simulink library "LopesDevelopmentLibrary"  (R2015b)
settings: Solver=ode45  StartTime=0.0  StopTime=10.0  RelTol=1e-3
values from neighbouring files (symbols this model uses):
  d2r = @(d) d*(pi/180)    [LopesDevelopmentLibrary_LoadParameters.m]
  ts = LopesParams.ts    [LopesDevelopmentLibrary_LoadParameters.m]
undefined symbols (not defined in the file or in its folder): anyParameterChanged, DiscIntNeverNeededParam, gcbh, LAP, LHF, LKF, LopesParams, macaddr, mxpcnetworkconfig, mxpcrtudprx, mxpcrtudptx, patientParametersChanged, port, PX, PZ, RAP, RHF, RKF, SelectorLOPESInSize, StrideTime_s, Time
undefined symbols (not defined in the file): LopesParamsSendDataArrayLen
libraries: LopesDevelopmentLibrary x327, simulink x100, dspmtrx3 x49, xpciplib x6, xpcnetworkbufferlib x5, dspsigops x4, dspstat3 x3, xpcethernetlib x2, visionstatistics x2, xpcseriallib x2, LopesDevelopmentLibraryTest x1, nmc x1
(part 5 of 12)

== system LopesDevelopmentLibrary/GaitGeneration/CalculateReferenceStiffnesses/RHA1 ==
  General_GuidanceForce : Inport
  breaks : Inport  Port=2
  phase : Inport  Port=3
  WeightShift_GuidanceForce : Inport  Port=4
  Circumduction_GuidanceForce : Inport  Port=5
  CalculateStiffnessForOneJoint : LopesDevelopmentLibrary/BlocksForInternalUse/GaitGeneration/CalculateStiffnessForOneJoint
  Constant : Constant  Value=LopesParams.GaitData.StiffnessParameters.HA_WeightShift
  Constant1 : Constant  Value=LopesParams.GaitData.StiffnessParameters.HA_Circumduction
  Mux : Mux  Inputs=2
  Mux1 : Mux  Inputs=2
  TrajectoryOfInfluence : LopesDevelopmentLibrary/BlocksForInternalUse/GaitGeneration/TrajectoryOfInfluence
  TrajectoryOfInfluence1 : LopesDevelopmentLibrary/BlocksForInternalUse/GaitGeneration/TrajectoryOfInfluence
  Stiffness_pct : Outport
  wires:
  Mux1/1 -> CalculateStiffnessForOneJoint/3
  Mux/1 -> CalculateStiffnessForOneJoint/2
  Circumduction_GuidanceForce/1 -> Mux1/2
  TrajectoryOfInfluence1/1 -> Mux/2
  TrajectoryOfInfluence/1 -> Mux/1
  phase/1 -> TrajectoryOfInfluence1/3, TrajectoryOfInfluence/3
  breaks/1 -> TrajectoryOfInfluence1/2, TrajectoryOfInfluence/2
  Constant/1 -> TrajectoryOfInfluence/1
  WeightShift_GuidanceForce/1 -> Mux1/1
  Constant1/1 -> TrajectoryOfInfluence1/1
  General_GuidanceForce/1 -> CalculateStiffnessForOneJoint/1
  CalculateStiffnessForOneJoint/1 -> Stiffness_pct/1

== system LopesDevelopmentLibrary/GaitGeneration/CalculateReferenceStiffnesses/RHF ==
  General_GuidanceForce : Inport
  breaks : Inport  Port=2
  phase : Inport  Port=3
  FootPlacement_GuidanceForce : Inport  Port=4
  StepLength_GuidanceForce : Inport  Port=5
  CalculateStiffnessForOneJoint : LopesDevelopmentLibrary/BlocksForInternalUse/GaitGeneration/CalculateStiffnessForOneJoint
  Constant : Constant  Value=LopesParams.GaitData.StiffnessParameters.HF_FootPlacement
  Constant1 : Constant  Value=LopesParams.GaitData.StiffnessParameters.HF_StepLength
  Mux : Mux  Inputs=2
  Mux1 : Mux  Inputs=2
  TrajectoryOfInfluence : LopesDevelopmentLibrary/BlocksForInternalUse/GaitGeneration/TrajectoryOfInfluence
  TrajectoryOfInfluence1 : LopesDevelopmentLibrary/BlocksForInternalUse/GaitGeneration/TrajectoryOfInfluence
  Stiffness_pct : Outport
  wires:
  phase/1 -> TrajectoryOfInfluence1/3, TrajectoryOfInfluence/3
  breaks/1 -> TrajectoryOfInfluence1/2, TrajectoryOfInfluence/2
  Constant/1 -> TrajectoryOfInfluence/1
  FootPlacement_GuidanceForce/1 -> Mux1/1
  CalculateStiffnessForOneJoint/1 -> Stiffness_pct/1
  Constant1/1 -> TrajectoryOfInfluence1/1
  StepLength_GuidanceForce/1 -> Mux1/2
  TrajectoryOfInfluence/1 -> Mux/1
  TrajectoryOfInfluence1/1 -> Mux/2
  Mux/1 -> CalculateStiffnessForOneJoint/2
  Mux1/1 -> CalculateStiffnessForOneJoint/3
  General_GuidanceForce/1 -> CalculateStiffnessForOneJoint/1

== system LopesDevelopmentLibrary/GaitGeneration/CalculateReferenceStiffnesses/RKF ==
  General_GuidanceForce : Inport
  breaks : Inport  Port=2
  phase : Inport  Port=3
  StepHeight_GuidanceForce : Inport  Port=4
  StabilityInStance_GuidanceForce : Inport  Port=5
  FootPlacement_GuidanceForce : Inport  Port=6
  CalculateStiffnessForOneJoint : LopesDevelopmentLibrary/BlocksForInternalUse/GaitGeneration/CalculateStiffnessForOneJoint
  Constant : Constant  Value=LopesParams.GaitData.StiffnessParameters.KF_StepHeight
  Constant1 : Constant  Value=LopesParams.GaitData.StiffnessParameters.KF_StabilityStance
  Constant2 : Constant  Value=LopesParams.GaitData.StiffnessParameters.KF_FootPlacement
  Mux : Mux  Inputs=3
  Mux1 : Mux  Inputs=3
  TrajectoryOfInfluence : LopesDevelopmentLibrary/BlocksForInternalUse/GaitGeneration/TrajectoryOfInfluence
  TrajectoryOfInfluence1 : LopesDevelopmentLibrary/BlocksForInternalUse/GaitGeneration/TrajectoryOfInfluence
  TrajectoryOfInfluence2 : LopesDevelopmentLibrary/BlocksForInternalUse/GaitGeneration/TrajectoryOfInfluence
  Stiffness_pct : Outport
  wires:
  StabilityInStance_GuidanceForce/1 -> Mux1/2
  Constant1/1 -> TrajectoryOfInfluence1/1
  TrajectoryOfInfluence1/1 -> Mux/2
  TrajectoryOfInfluence/1 -> Mux/1
  StepHeight_GuidanceForce/1 -> Mux1/1
  Constant/1 -> TrajectoryOfInfluence/1
  breaks/1 -> TrajectoryOfInfluence/2, TrajectoryOfInfluence2/2, TrajectoryOfInfluence1/2
  phase/1 -> TrajectoryOfInfluence/3, TrajectoryOfInfluence2/3, TrajectoryOfInfluence1/3
  FootPlacement_GuidanceForce/1 -> Mux1/3
  Constant2/1 -> TrajectoryOfInfluence2/1
  TrajectoryOfInfluence2/1 -> Mux/3
  CalculateStiffnessForOneJoint/1 -> Stiffness_pct/1
  Mux/1 -> CalculateStiffnessForOneJoint/2
  Mux1/1 -> CalculateStiffnessForOneJoint/3
  General_GuidanceForce/1 -> CalculateStiffnessForOneJoint/1

== system LopesDevelopmentLibrary/GaitGeneration/GaitParameters/AssignChangedElements ==
  note: This block checks whether any of the parameters changed during
      | this sampletime, and assigns the correct values to the anyParameterChanged
      | and patientParametersChanged bus elements.
  BusIn : Inport
  PatientParametersChanged : Inport  Port=2
  AnyChanged : LopesDevelopmentLibrary/Various/AnyChanged
  Bus Assignment : BusAssignment  AssignedSignals=patientParametersChanged,anyParameterChanged
  Bus Selector : BusSelector  OutputSignals=Patient,General,WeightShift,LeftStepHeight,RightStepHeight,LeftCircumduction,RightCircumduction,LeftStabilityStance,RightStabilityStance,LeftPrepositioning,RightPrepositioning,LeftSteplength,RightSteplength  OutputAsBus=on
  Data Type Conversion2 : DataTypeConversion
  Logical Operator : Logic  Operator=OR  AllPortsSameDT=off  OutDataTypeStr=boolean
  BusOut : Outport
  Changed : Outport  Port=2
  wires:
  Data Type Conversion2/1 -> Changed/1
  Bus Assignment/1 -> BusOut/1
  Bus Selector/1 -> AnyChanged/1
  PatientParametersChanged/1 -> Logical Operator/1, Bus Assignment/2
  BusIn/1 -> Bus Selector/1, Bus Assignment/1
  Logical Operator/1 -> Bus Assignment/3, Data Type Conversion2/1
  AnyChanged/1 -> Logical Operator/2

== system LopesDevelopmentLibrary/GaitGeneration/GaitParameters/Circumduction ==

== system LopesDevelopmentLibrary/GaitGeneration/GaitParameters/General ==

== system LopesDevelopmentLibrary/GaitGeneration/GaitParameters/Prepositioning ==

== system LopesDevelopmentLibrary/GaitGeneration/GaitParameters/Pushoff ==

== system LopesDevelopmentLibrary/GaitGeneration/GaitParameters/RateLimitCircumduction ==
  GeneralGF : Inport
  In2 : Inport  Port=2
  In3 : Inport  Port=3
  In4 : Inport  Port=4
  In5 : Inport  Port=5
  In6 : Inport  Port=6
  In7 : Inport  Port=7
  Bus Creator1 : BusCreator  Inputs=2
  Bus Creator2 : BusCreator  Inputs=2
  Rate Limiter : RateLimiter  RisingSlewLimit=100  FallingSlewLimit=-100  SampleTimeMode=inherited
  Rate Limiter1 : RateLimiter  RisingSlewLimit=50  FallingSlewLimit=-50  SampleTimeMode=inherited
  Rate Limiter2 : RateLimiter  RisingSlewLimit=50  FallingSlewLimit=-50  SampleTimeMode=inherited
  Rate Limiter7 : RateLimiter  RisingSlewLimit=100  FallingSlewLimit=-100  SampleTimeMode=inherited
  Switch : Switch  Criteria=u2 ~= 0
  Switch1 : Switch  Criteria=u2 ~= 0
  Left : Outport
  Right : Outport  Port=2
  wires:
  Bus Creator1/1 -> Left/1
  Rate Limiter1/1 -> Bus Creator1/2  "Circumduction_pct"
  Rate Limiter/1 -> Bus Creator1/1  "GuidanceForce_pct"
  Switch1/1 -> Rate Limiter7/1
  In2/1 -> Switch/2
  In6/1 -> Switch1/1
  In3/1 -> Switch/1
  In5/1 -> Switch1/2
  In7/1 -> Rate Limiter2/1
  Switch/1 -> Rate Limiter/1  "GuidanceForce_pct"
  In4/1 -> Rate Limiter1/1
  GeneralGF/1 -> Switch/3, Switch1/3
  Rate Limiter2/1 -> Bus Creator2/2  "Circumduction_pct"
  Rate Limiter7/1 -> Bus Creator2/1  "GuidanceForce_pct"
  Bus Creator2/1 -> Right/1

== system LopesDevelopmentLibrary/GaitGeneration/GaitParameters/RateLimitGeneral ==
  In1 : Inport
  In2 : Inport  Port=2
  In3 : Inport  Port=3
  Bus Creator1 : BusCreator  Inputs=3
  ConvertToKm_h : Gain  Gain=3.6
  Rate Limiter1 : RateLimiter  RisingSlewLimit=50  FallingSlewLimit=-50  SampleTimeMode=inherited
  Rate Limiter2 : RateLimiter  RisingSlewLimit=0.1  FallingSlewLimit=-0.1  SampleTimeMode=inherited
  Rate Limiter3 : RateLimiter  RisingSlewLimit=20  FallingSlewLimit=-20  SampleTimeMode=inherited
  km_h : Outport
  General : Outport  Port=2
  wires:
  Bus Creator1/1 -> General/1  "General"
  In3/1 -> Rate Limiter1/1
  In2/1 -> Rate Limiter3/1
  In1/1 -> ConvertToKm_h/1, Rate Limiter2/1
  ConvertToKm_h/1 -> km_h/1
  Rate Limiter2/1 -> Bus Creator1/1  "WalkingVelocity_m_s"
  Rate Limiter3/1 -> Bus Creator1/2  "GuidanceForce_pct"
  Rate Limiter1/1 -> Bus Creator1/3  "HipExtensionOffset"

== system LopesDevelopmentLibrary/GaitGeneration/GaitParameters/RateLimitPrepositioning ==
  GeneralGF : Inport
  In2 : Inport  Port=2
  In3 : Inport  Port=3
  In4 : Inport  Port=4
  In1 : Inport  Port=5
  In5 : Inport  Port=6
  In6 : Inport  Port=7
  In7 : Inport  Port=8
  In8 : Inport  Port=9
  Bus Creator1 : BusCreator  Inputs=3
  Bus Creator2 : BusCreator  Inputs=3
  Rate Limiter : RateLimiter  RisingSlewLimit=100  FallingSlewLimit=-100  SampleTimeMode=inherited
  Rate Limiter{1..4} (4 alike) : RateLimiter  RisingSlewLimit=50  FallingSlewLimit=-50  SampleTimeMode=inherited
  Rate Limiter7 : RateLimiter  RisingSlewLimit=100  FallingSlewLimit=-100  SampleTimeMode=inherited
  Switch : Switch  Criteria=u2 ~= 0
  Switch1 : Switch  Criteria=u2 ~= 0
  Left : Outport
  Right : Outport  Port=2
  wires:
  Bus Creator1/1 -> Left/1
  Rate Limiter1/1 -> Bus Creator1/2  "KneeFlexion_pct"
  Rate Limiter/1 -> Bus Creator1/1  "GuidanceForce_pct"
  Switch1/1 -> Rate Limiter7/1
  In2/1 -> Switch/2
  In6/1 -> Switch1/1
  In3/1 -> Switch/1
  In5/1 -> Switch1/2
  In7/1 -> Rate Limiter2/1
  Switch/1 -> Rate Limiter/1  "GuidanceForce_pct"
  In4/1 -> Rate Limiter1/1
  GeneralGF/1 -> Switch/3, Switch1/3
  Rate Limiter2/1 -> Bus Creator2/2  "KneeFlexion_pct"
  Rate Limiter7/1 -> Bus Creator2/1  "GuidanceForce_pct"
  Bus Creator2/1 -> Right/1
  Rate Limiter3/1 -> Bus Creator1/3  "AnkleDorsiflexion_pct"
  In1/1 -> Rate Limiter3/1
  Rate Limiter4/1 -> Bus Creator2/3  "AnkleDorsiflexion_pct"
  In8/1 -> Rate Limiter4/1

== system LopesDevelopmentLibrary/GaitGeneration/GaitParameters/RateLimitPushoff ==
  GeneralGF : Inport
  In2 : Inport  Port=2
  In3 : Inport  Port=3
  In4 : Inport  Port=4
  In1 : Inport  Port=5
  In5 : Inport  Port=6
  In6 : Inport  Port=7
  In7 : Inport  Port=8
  In8 : Inport  Port=9
  Bus Creator1 : BusCreator  Inputs=3
  Bus Creator2 : BusCreator  Inputs=3
  Rate Limiter : RateLimiter  RisingSlewLimit=100  FallingSlewLimit=-100  SampleTimeMode=inherited
  Rate Limiter1 : RateLimiter  RisingSlewLimit=50  FallingSlewLimit=-50  SampleTimeMode=inherited
  Rate Limiter2 : RateLimiter  RisingSlewLimit=50  FallingSlewLimit=-50  SampleTimeMode=inherited
  Rate Limiter3 : RateLimiter  RisingSlewLimit=10  FallingSlewLimit=-10  SampleTimeMode=inherited
  Rate Limiter4 : RateLimiter  RisingSlewLimit=10  FallingSlewLimit=-10  SampleTimeMode=inherited
  Rate Limiter7 : RateLimiter  RisingSlewLimit=100  FallingSlewLimit=-100  SampleTimeMode=inherited
  Switch : Switch  Criteria=u2 ~= 0
  Switch1 : Switch  Criteria=u2 ~= 0
  Left : Outport
  Right : Outport  Port=2
  wires:
  In8/1 -> Rate Limiter4/1
  Rate Limiter4/1 -> Bus Creator2/3  "Timing_pct"
  In1/1 -> Rate Limiter3/1
  Rate Limiter3/1 -> Bus Creator1/3  "Timing_pct"
  Bus Creator2/1 -> Right/1
  Rate Limiter7/1 -> Bus Creator2/1  "GuidanceForce_pct"
  Rate Limiter2/1 -> Bus Creator2/2  "HipExtension_pct"
  GeneralGF/1 -> Switch1/3, Switch/3
  In4/1 -> Rate Limiter1/1
  Switch/1 -> Rate Limiter/1  "GuidanceForce_pct"
  In7/1 -> Rate Limiter2/1
  In5/1 -> Switch1/2
  In3/1 -> Switch/1
  In6/1 -> Switch1/1
  In2/1 -> Switch/2
  Switch1/1 -> Rate Limiter7/1
  Rate Limiter/1 -> Bus Creator1/1  "GuidanceForce_pct"
  Rate Limiter1/1 -> Bus Creator1/2  "HipExtension_pct"
  Bus Creator1/1 -> Left/1

== system LopesDevelopmentLibrary/GaitGeneration/GaitParameters/RateLimitStabilityStance ==
  GeneralGF : Inport
  In2 : Inport  Port=2
  In3 : Inport  Port=3
  In4 : Inport  Port=4
  In5 : Inport  Port=5
  In6 : Inport  Port=6
  In7 : Inport  Port=7
  Bus Creator1 : BusCreator  Inputs=2
  Bus Creator2 : BusCreator  Inputs=2
  Rate Limiter : RateLimiter  RisingSlewLimit=100  FallingSlewLimit=-100  SampleTimeMode=inherited
  Rate Limiter1 : RateLimiter  RisingSlewLimit=50  FallingSlewLimit=-50  SampleTimeMode=inherited
  Rate Limiter2 : RateLimiter  RisingSlewLimit=50  FallingSlewLimit=-50  SampleTimeMode=inherited
  Rate Limiter7 : RateLimiter  RisingSlewLimit=100  FallingSlewLimit=-100  SampleTimeMode=inherited
  Switch : Switch  Criteria=u2 ~= 0
  Switch1 : Switch  Criteria=u2 ~= 0
  Left : Outport
  Right : Outport  Port=2
  wires:
  Bus Creator2/1 -> Right/1
  Rate Limiter7/1 -> Bus Creator2/1  "GuidanceForce_pct"
  Rate Limiter2/1 -> Bus Creator2/2  "KneeFlexion_pct"
  GeneralGF/1 -> Switch1/3, Switch/3
  In4/1 -> Rate Limiter1/1
  Switch/1 -> Rate Limiter/1  "GuidanceForce_pct"
  In7/1 -> Rate Limiter2/1
  In5/1 -> Switch1/2
  In3/1 -> Switch/1
  In6/1 -> Switch1/1
  In2/1 -> Switch/2
  Switch1/1 -> Rate Limiter7/1
  Rate Limiter/1 -> Bus Creator1/1  "GuidanceForce_pct"
  Rate Limiter1/1 -> Bus Creator1/2  "KneeFlexion_pct"
  Bus Creator1/1 -> Left/1

== system LopesDevelopmentLibrary/GaitGeneration/GaitParameters/RateLimitStepHeight ==
  GeneralGF : Inport
  In2 : Inport  Port=2
  In3 : Inport  Port=3
  In1 : Inport  Port=4
  In4 : Inport  Port=5
  In5 : Inport  Port=6
  In6 : Inport  Port=7
  In8 : Inport  Port=8
  In7 : Inport  Port=9
  Bus Creator1 : BusCreator  Inputs=3
  Bus Creator2 : BusCreator  Inputs=3
  Rate Limiter : RateLimiter  RisingSlewLimit=100  FallingSlewLimit=-100  SampleTimeMode=inherited
  Rate Limiter1 : RateLimiter  RisingSlewLimit=50  FallingSlewLimit=-50  SampleTimeMode=inherited
  Rate Limiter2 : RateLimiter  RisingSlewLimit=50  FallingSlewLimit=-50  SampleTimeMode=inherited
  Rate Limiter3 : RateLimiter  RisingSlewLimit=100  FallingSlewLimit=-100  SampleTimeMode=inherited
  Rate Limiter4 : RateLimiter  RisingSlewLimit=50  FallingSlewLimit=-50  SampleTimeMode=inherited
  Rate Limiter7 : RateLimiter  RisingSlewLimit=100  FallingSlewLimit=-100  SampleTimeMode=inherited
  Switch : Switch  Criteria=u2 ~= 0
  Switch1 : Switch  Criteria=u2 ~= 0
  Left : Outport
  Right : Outport  Port=2
  wires:
  Bus Creator2/1 -> Right/1
  Rate Limiter7/1 -> Bus Creator2/1  "GuidanceForce_pct"
  Rate Limiter2/1 -> Bus Creator2/3  "KneeFlexion_pct"
  GeneralGF/1 -> Switch/3, Switch1/3
  In4/1 -> Rate Limiter1/1
  Switch/1 -> Rate Limiter/1  "GuidanceForce_pct"
  In7/1 -> Rate Limiter2/1
  In5/1 -> Switch1/2
  In3/1 -> Switch/1
  In6/1 -> Switch1/1
  In2/1 -> Switch/2
  Switch1/1 -> Rate Limiter7/1
  Rate Limiter/1 -> Bus Creator1/1  "GuidanceForce_pct"
  Rate Limiter1/1 -> Bus Creator1/3  "KneeFlexion_pct"
  Bus Creator1/1 -> Left/1
  Rate Limiter3/1 -> Bus Creator1/2  "AnkleDorsiflexion_pct"
  In1/1 -> Rate Limiter3/1
  Rate Limiter4/1 -> Bus Creator2/2  "AnkleDorsiflexion_pct"
  In8/1 -> Rate Limiter4/1

== system LopesDevelopmentLibrary/GaitGeneration/GaitParameters/RateLimitStepLength ==
  GeneralGF : Inport
  In2 : Inport  Port=2
  In3 : Inport  Port=3
  In4 : Inport  Port=4
  Bus Creator1 : BusCreator  Inputs=2
  Rate Limiter : RateLimiter  RisingSlewLimit=100  FallingSlewLimit=-100  SampleTimeMode=inherited
  Rate Limiter1 : RateLimiter  RisingSlewLimit=5  FallingSlewLimit=-5  SampleTimeMode=inherited
  Switch : Switch  Criteria=u2 ~= 0
  StepLength : Outport
  wires:
  GeneralGF/1 -> Switch/3
  In4/1 -> Rate Limiter1/1
  Switch/1 -> Rate Limiter/1  "GuidanceForce_pct"
  In3/1 -> Switch/1
  In2/1 -> Switch/2
  Rate Limiter/1 -> Bus Creator1/1  "GuidanceForce_pct"
  Rate Limiter1/1 -> Bus Creator1/2  "StepLength_pct"
  Bus Creator1/1 -> StepLength/1

== system LopesDevelopmentLibrary/GaitGeneration/GaitParameters/RateLimitWeightShift ==
  GeneralGF : Inport
  In2 : Inport  Port=2
  In3 : Inport  Port=3
  In4 : Inport  Port=4
  In5 : Inport  Port=5
  In6 : Inport  Port=6
  In7 : Inport  Port=7
  In8 : Inport  Port=8
  In9 : Inport  Port=9
  Bus Creator1 : BusCreator  Inputs=7
  Rate Limiter : RateLimiter  RisingSlewLimit=50  FallingSlewLimit=-50  SampleTimeMode=inherited
  Rate Limiter1 : RateLimiter  RisingSlewLimit=50  FallingSlewLimit=-50  SampleTimeMode=inherited
  Rate Limiter2 : RateLimiter  RisingSlewLimit=50  FallingSlewLimit=-50  SampleTimeMode=inherited
  Rate Limiter3 : RateLimiter  RisingSlewLimit=15  FallingSlewLimit=-15  SampleTimeMode=inherited
  Rate Limiter4 : RateLimiter  RisingSlewLimit=15  FallingSlewLimit=-15  SampleTimeMode=inherited
  Rate Limiter5 : RateLimiter  RisingSlewLimit=15  FallingSlewLimit=-15  SampleTimeMode=inherited
  Rate Limiter6 : RateLimiter  RisingSlewLimit=20  FallingSlewLimit=-20  SampleTimeMode=inherited
  Switch : Switch  Criteria=u2 ~= 0
  Out1 : Outport
  wires:
  In3/1 -> Switch/1
  Switch/1 -> Rate Limiter/1  "GuidanceForce_pct"
  In7/1 -> Rate Limiter4/1
  In8/1 -> Rate Limiter5/1
  In9/1 -> Rate Limiter6/1
  In4/1 -> Rate Limiter1/1
  In5/1 -> Rate Limiter2/1
  In6/1 -> Rate Limiter3/1
  GeneralGF/1 -> Switch/3
  Rate Limiter5/1 -> Bus Creator1/6  "DurationRight_pct"
  Rate Limiter/1 -> Bus Creator1/1  "GuidanceForce_pct"
  Rate Limiter4/1 -> Bus Creator1/5  "DurationLeft_pct"
  Rate Limiter3/1 -> Bus Creator1/4  "Timing_pct"
  Rate Limiter1/1 -> Bus Creator1/2  "AmplitudeLeft_pct"
  Rate Limiter6/1 -> Bus Creator1/7  "StepWidth_pct"
  Bus Creator1/1 -> Out1/1
  Rate Limiter2/1 -> Bus Creator1/3  "AmplitudeRight_pct"
  In2/1 -> Switch/2

== system LopesDevelopmentLibrary/GaitGeneration/GaitParameters/StabilityInStance ==

== system LopesDevelopmentLibrary/GaitGeneration/GaitParameters/StepHeight ==

== system LopesDevelopmentLibrary/GaitGeneration/GaitParameters/StepLength ==

== system LopesDevelopmentLibrary/GaitGeneration/GaitParameters/WeightShift ==

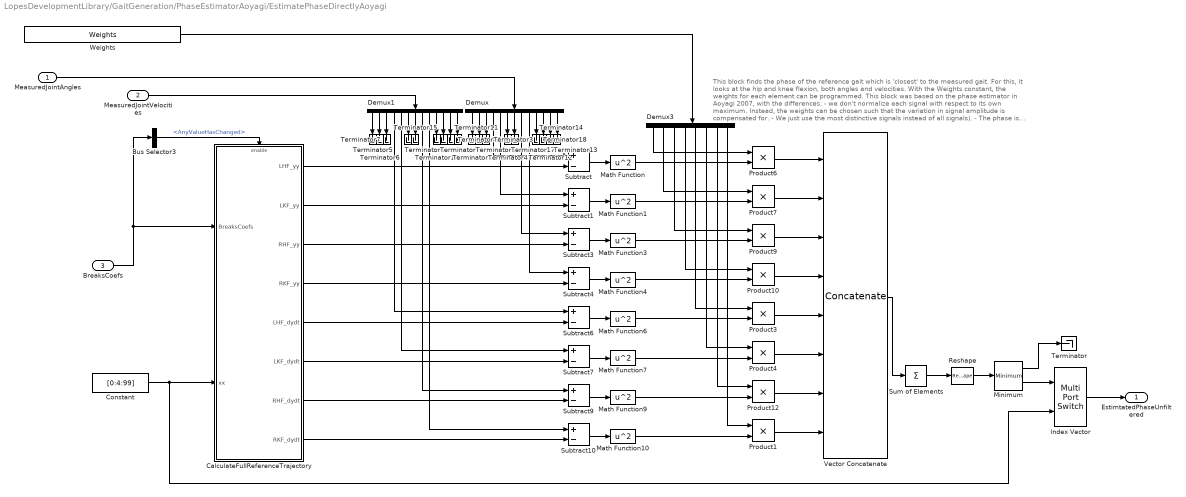
== system LopesDevelopmentLibrary/GaitGeneration/PhaseEstimatorAoyagi/EstimatePhaseDirectlyAoyagi ==
  note: This block finds the phase of the reference gait which is 'closest' to the
      | measured gait. For this, it looks at the hip and knee flexion,
      | both angles and velocities. With the Weights constant, the weights for each element
      | can be programmed.
      | This block was based on the phase estimator in Aoyagi 2007, with the differences:
      | - we don't normalize each signal with respect to its own maximum. Instead, the weights
      | can be chosen such that the variation in signal amplitude is compensated for.
      | - We just use the most distinctive signals instead of all signals).
      | - The phase is expressed in percent  [0,100) instead of [0,1).
  MeasuredJointAngles : Inport
  MeasuredJointVelocities : Inport  Port=2
  BreaksCoefs : Inport  Port=3
  Bus Selector3 : BusSelector  OutputSignals=AnyValueHasChanged
  CalculateFullReferenceTrajectory : Subsystem
  Constant : Constant  Value=[0:4:99]
  Demux : Demux  Outputs=13
  Demux1 : Demux  Outputs=13
  Demux3 : Demux  Outputs=8
  Index Vector : MultiPortSwitch  Inputs=1
  Math Function{,1,3..4,6..7,9..10} (8 alike) : Math  Operator=square  SaturateOnIntegerOverflow=on
  Minimum : dspstat3/Minimum  fcn=Value and Index  reset=None  InputProcessing=Columns as channels (frame based)  indexBase=One  operateOver=Each column  Dimension=1  operation=minimum  roiEnable=off  roiType=Rectangles  roiPortion=Entire ROI  roiOutput=Individual statistics for each ROI  roiFlag=off  roundingMode=Floor  overflowMode=off
  Product{1,3..4,6..7,9..10,12} (8 alike) : Product  RndMeth=Zero
  Reshape : Reshape
  Subtract{,1,3..4,6..7,9..10} (8 alike) : Sum  Inputs=+-
  Sum of Elements : Sum  Inputs=+  CollapseMode=Specified dimension  CollapseDim=2
  Terminator{,1..18} (19 alike) : Terminator
  Vector Concatenate : Concatenate  NumInputs=8  Mode=Multidimensional array  ConcatenateDimension=2
  Weights : Constant  Value=Weights
  EstimtatedPhaseUnfiltered : Outport
  wires:
  Demux/6 -> Terminator4/1
  Demux/3 -> Terminator3/1
  Demux/2 -> Terminator2/1
  Demux/1 -> Terminator1/1
  Demux1/1 -> Terminator5/1
  Demux1/2 -> Terminator6/1
  Demux1/3 -> Terminator7/1
  Demux1/6 -> Terminator8/1
  Minimum/1 -> Terminator/1
  Demux/5 -> Subtract1/1
  Demux/4 -> Subtract/1
  Constant/1 -> Index Vector/2, CalculateFullReferenceTrajectory/2(xx)
  MeasuredJointAngles/1 -> Demux/1
  BreaksCoefs/1 -> Bus Selector3/1, CalculateFullReferenceTrajectory/1(BreaksCoefs)
  Index Vector/1 -> EstimtatedPhaseUnfiltered/1
  Demux/8 -> Subtract3/1
  Demux/9 -> Subtract4/1
  Subtract/1 -> Math Function/1
  Subtract1/1 -> Math Function1/1
  Subtract3/1 -> Math Function3/1
  Subtract4/1 -> Math Function4/1
  Math Function/1 -> Product6/2
  Math Function1/1 -> Product7/2
  Math Function3/1 -> Product9/2
  Math Function4/1 -> Product10/2
  Weights/1 -> Demux3/1
  Product7/1 -> Vector Concatenate/2
  Product6/1 -> Vector Concatenate/1
  Product9/1 -> Vector Concatenate/3
  Product10/1 -> Vector Concatenate/4
  Vector Concatenate/1 -> Sum of Elements/1
  Sum of Elements/1 -> Reshape/1
  Minimum/2 -> Index Vector/1
  MeasuredJointVelocities/1 -> Demux1/1
  Subtract6/1 -> Math Function6/1
  Subtract7/1 -> Math Function7/1
  Subtract9/1 -> Math Function9/1
  Subtract10/1 -> Math Function10/1
  Demux1/4 -> Subtract6/1
  Demux1/5 -> Subtract7/1
  Demux1/8 -> Subtract9/1
  Demux1/9 -> Subtract10/1
  Math Function6/1 -> Product3/2
  Math Function7/1 -> Product4/2
  Math Function9/1 -> Product12/2
  Math Function10/1 -> Product1/2
  Product4/1 -> Vector Concatenate/6
  Product3/1 -> Vector Concatenate/5
  Product12/1 -> Vector Concatenate/7
  Product1/1 -> Vector Concatenate/8
  Reshape/1 -> Minimum/1
  CalculateFullReferenceTrajectory/1(LHF_yy) -> Subtract/2
  CalculateFullReferenceTrajectory/2(LKF_yy) -> Subtract1/2
  CalculateFullReferenceTrajectory/3(RHF_yy) -> Subtract3/2
  CalculateFullReferenceTrajectory/4(RKF_yy) -> Subtract4/2
  CalculateFullReferenceTrajectory/5(LHF_dydt) -> Subtract6/2
  CalculateFullReferenceTrajectory/6(LKF_dydt) -> Subtract7/2
  CalculateFullReferenceTrajectory/7(RHF_dydt) -> Subtract9/2
  CalculateFullReferenceTrajectory/8(RKF_dydt) -> Subtract10/2
  Bus Selector3/1 -> CalculateFullReferenceTrajectory/Enable  "<AnyValueHasChanged>"
  Demux3/1 -> Product6/1
  Demux3/2 -> Product7/1
  Demux3/3 -> Product9/1
  Demux3/4 -> Product10/1
  Demux3/5 -> Product3/1
  Demux3/6 -> Product4/1
  Demux3/7 -> Product12/1
  Demux3/8 -> Product1/1
  Demux1/7 -> Terminator15/1
  Demux1/10 -> Terminator16/1
  Demux/7 -> Terminator17/1
  Demux1/11 -> Terminator9/1
  Demux1/12 -> Terminator10/1
  Demux1/13 -> Terminator11/1
  Demux/10 -> Terminator18/1
  Demux/11 -> Terminator14/1
  Demux/12 -> Terminator12/1
  Demux/13 -> Terminator13/1

== system LopesDevelopmentLibrary/GaitGeneration/PhaseEstimatorAoyagi/PhaseFilterAoyagi ==
  note: This filter is based on the filter described in Aoyagi 2007.
      | It differs on the following points:
      | - Range [0,100) %, not [0,1) scale.
      | - Different implementation of wrap around integration (Aoyagi uses a resettable integrator; I use a mod 100)
      | - AoyagiFilterGain should be the same as in the paper (the error is 100 times larger than Aoyagi's, but so is
      |    the range of the integration). I found however that 2.5 for a gain [Aoyagi 2007] is quite low.
      | - In the figure in the paper no saturation is shown, but in the text they tell that there is saturation. I use it
      |    here too (so that phase cannot go backwards and cannot go rise too fast).
  EstimatedPhaseUnfiltered : Inport
  ReferenceStrideTime : Inport  Port=2
  ResetHighActive : Inport  Port=3
  AoyagiFilterGain : Gain  Gain=AoyagiFilterGain
  CalculateStridesPerSec : Math  Operator=reciprocal  SaturateOnIntegerOverflow=on
  Integrator : Integrator  ExternalReset=level
  PhaseWrapper : LopesDevelopmentLibrary/Various/PhaseWrapper
  Saturation : Saturate  UpperLimit=300  LowerLimit=0
  Sum : Sum  Inputs=|+-
  Sum1 : Sum  Inputs=++|
  ToPercentPerSec : Gain  Gain=100
  Wrap_Min50_Plus50 : Subsystem
  EstimatedPhase : Outport
  EstimatedPhaseRate : Outport  Port=2
  wires:
  ReferenceStrideTime/1 -> CalculateStridesPerSec/1
  Sum/1 -> Wrap_Min50_Plus50/1(In)
  Saturation/1 -> EstimatedPhaseRate/1, Integrator/1
  Wrap_Min50_Plus50/1(Out) -> AoyagiFilterGain/1
  CalculateStridesPerSec/1 -> ToPercentPerSec/1
  PhaseWrapper/1 -> EstimatedPhase/1, Sum/2
  ToPercentPerSec/1 -> Sum1/1
  AoyagiFilterGain/1 -> Sum1/2
  Sum1/1 -> Saturation/1
  EstimatedPhaseUnfiltered/1 -> Sum/1
  Integrator/1 -> PhaseWrapper/1
  ResetHighActive/1 -> Integrator/2

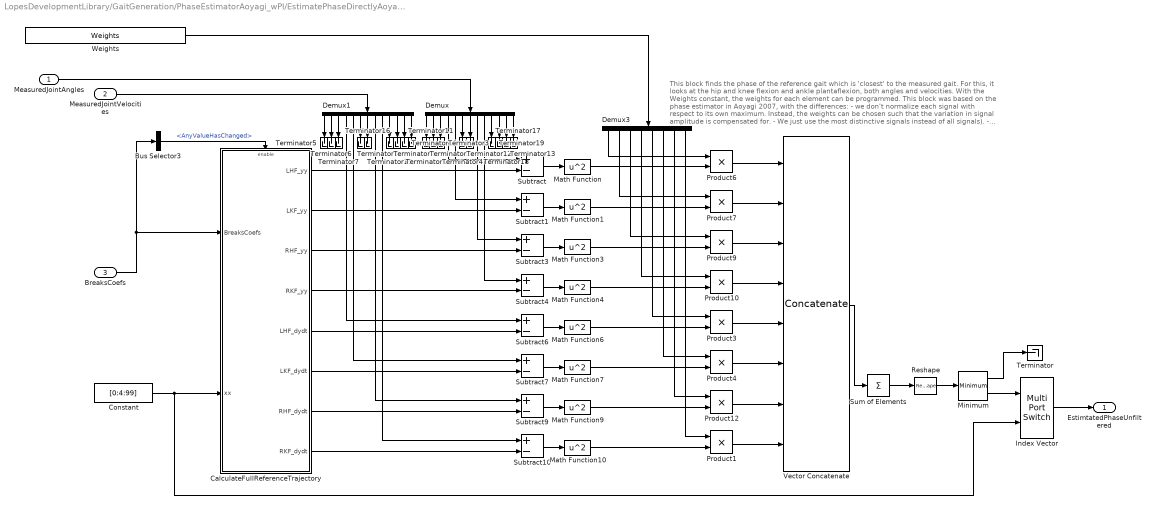
== system LopesDevelopmentLibrary/GaitGeneration/PhaseEstimatorAoyagi_wPI/EstimatePhaseDirectlyAoyagi ==
  note: This block finds the phase of the reference gait which is 'closest' to the
      | measured gait. For this, it looks at the hip and knee flexion and ankle plantaflexion,
      | both angles and velocities. With the Weights constant, the weights for each element
      | can be programmed.
      | This block was based on the phase estimator in Aoyagi 2007, with the differences:
      | - we don't normalize each signal with respect to its own maximum. Instead, the weights
      | can be chosen such that the variation in signal amplitude is compensated for.
      | - We just use the most distinctive signals instead of all signals).
      | - The phase is expressed in percent  [0,100) instead of [0,1).
  MeasuredJointAngles : Inport
  MeasuredJointVelocities : Inport  Port=2
  BreaksCoefs : Inport  Port=3
  Bus Selector3 : BusSelector  OutputSignals=AnyValueHasChanged
  CalculateFullReferenceTrajectory : Subsystem
  Constant : Constant  Value=[0:4:99]
  Demux : Demux  Outputs=13
  Demux1 : Demux  Outputs=13
  Demux3 : Demux  Outputs=8
  Index Vector : MultiPortSwitch  Inputs=1
  Math Function{,1,3..4,6..7,9..10} (8 alike) : Math  Operator=square  SaturateOnIntegerOverflow=on
  Minimum : dspstat3/Minimum  fcn=Value and Index  reset=None  InputProcessing=Columns as channels (frame based)  indexBase=One  operateOver=Each column  Dimension=1  operation=minimum  roiEnable=off  roiType=Rectangles  roiPortion=Entire ROI  roiOutput=Individual statistics for each ROI  roiFlag=off  roundingMode=Floor  overflowMode=off
  Product{1,3..4,6..7,9..10,12} (8 alike) : Product  RndMeth=Zero
  Reshape : Reshape
  Subtract{,1,3..4,6..7,9..10} (8 alike) : Sum  Inputs=+-
  Sum of Elements : Sum  Inputs=+  CollapseMode=Specified dimension  CollapseDim=2
  Terminator{,1..13,15..19} (19 alike) : Terminator
  Vector Concatenate : Concatenate  NumInputs=8  Mode=Multidimensional array  ConcatenateDimension=2
  Weights : Constant  Value=Weights
  EstimtatedPhaseUnfiltered : Outport
  wires:
  Demux3/8 -> Product1/1
  Demux3/7 -> Product12/1
  Demux3/6 -> Product4/1
  Demux3/5 -> Product3/1
  Demux3/4 -> Product10/1
  Demux3/3 -> Product9/1
  Demux3/2 -> Product7/1
  Demux3/1 -> Product6/1
  Bus Selector3/1 -> CalculateFullReferenceTrajectory/Enable  "<AnyValueHasChanged>"
  CalculateFullReferenceTrajectory/8(RKF_dydt) -> Subtract10/2
  CalculateFullReferenceTrajectory/7(RHF_dydt) -> Subtract9/2
  CalculateFullReferenceTrajectory/6(LKF_dydt) -> Subtract7/2
  CalculateFullReferenceTrajectory/5(LHF_dydt) -> Subtract6/2
  CalculateFullReferenceTrajectory/4(RKF_yy) -> Subtract4/2
  CalculateFullReferenceTrajectory/3(RHF_yy) -> Subtract3/2
  CalculateFullReferenceTrajectory/2(LKF_yy) -> Subtract1/2
  CalculateFullReferenceTrajectory/1(LHF_yy) -> Subtract/2
  Reshape/1 -> Minimum/1
  Product1/1 -> Vector Concatenate/8
  Product12/1 -> Vector Concatenate/7
  Product3/1 -> Vector Concatenate/5
  Product4/1 -> Vector Concatenate/6
  Math Function10/1 -> Product1/2
  Math Function9/1 -> Product12/2
  Math Function7/1 -> Product4/2
  Math Function6/1 -> Product3/2
  Demux1/9 -> Subtract10/1
  Demux1/8 -> Subtract9/1
  Demux1/5 -> Subtract7/1
  Demux1/4 -> Subtract6/1
  Subtract10/1 -> Math Function10/1
  Subtract9/1 -> Math Function9/1
  Subtract7/1 -> Math Function7/1
  Subtract6/1 -> Math Function6/1
  MeasuredJointVelocities/1 -> Demux1/1
  Minimum/2 -> Index Vector/1
  Sum of Elements/1 -> Reshape/1
  Vector Concatenate/1 -> Sum of Elements/1
  Product10/1 -> Vector Concatenate/4
  Product9/1 -> Vector Concatenate/3
  Product6/1 -> Vector Concatenate/1
  Product7/1 -> Vector Concatenate/2
  Weights/1 -> Demux3/1
  Math Function4/1 -> Product10/2
  Math Function3/1 -> Product9/2
  Math Function1/1 -> Product7/2
  Math Function/1 -> Product6/2
  Subtract4/1 -> Math Function4/1
  Subtract3/1 -> Math Function3/1
  Subtract1/1 -> Math Function1/1
  Subtract/1 -> Math Function/1
  Demux/9 -> Subtract4/1
  Demux/8 -> Subtract3/1
  Index Vector/1 -> EstimtatedPhaseUnfiltered/1
  BreaksCoefs/1 -> CalculateFullReferenceTrajectory/1(BreaksCoefs), Bus Selector3/1
  MeasuredJointAngles/1 -> Demux/1
  Constant/1 -> CalculateFullReferenceTrajectory/2(xx), Index Vector/2
  Demux/4 -> Subtract/1
  Demux/5 -> Subtract1/1
  Minimum/1 -> Terminator/1
  Demux1/6 -> Terminator8/1
  Demux1/3 -> Terminator7/1
  Demux1/2 -> Terminator6/1
  Demux1/1 -> Terminator5/1
  Demux/1 -> Terminator1/1
  Demux/2 -> Terminator2/1
  Demux/3 -> Terminator3/1
  Demux/6 -> Terminator4/1
  Demux1/10 -> Terminator15/1
  Demux1/11 -> Terminator9/1
  Demux/10 -> Terminator19/1
  Demux1/12 -> Terminator10/1
  Demux1/13 -> Terminator11/1
  Demux1/7 -> Terminator16/1
  Demux/13 -> Terminator13/1
  Demux/12 -> Terminator18/1
  Demux/11 -> Terminator17/1
  Demux/7 -> Terminator12/1

== system LopesDevelopmentLibrary/GaitGeneration/PhaseEstimatorAoyagi_wPI/PhaseFilterAoyagi ==
  note: This filter is based on the filter described in Aoyagi 2007.
      | It differs on the following points:
      | - Range [0,100) %, not [0,1) scale.
      | - Different implementation of wrap around integration (Aoyagi uses a resettable integrator; I use a mod 100)
      | - AoyagiFilterGain should be the same as in the paper (the error is 100 times larger than Aoyagi's, but so is
      |    the range of the integration). I found however that 2.5 for a gain [Aoyagi 2007] is quite low.
      | - In the figure in the paper no saturation is shown, but in the text they tell that there is saturation. I use it
      |    here too (so that phase cannot go backwards and cannot go rise too fast).
  note: "'PI-controller". Makes sure that the phase error will eventually
      | go to zero. Hopefully this will make the system better. However, the integral is
      | limited to -20..20 to prevent problems when a non-walking state is detected.
  EstimatedPhaseUnfiltered : Inport
  ReferenceStrideTime : Inport  Port=2
  ResetHighActive : Inport  Port=3
  AoyagiFilterGain : Gain  Gain=AoyagiFilterGain
  CalculateStridesPerSec : Math  Operator=reciprocal  SaturateOnIntegerOverflow=on
  Divide : Product  Inputs=/*
  Gain : Gain  Gain=3
  Gain1 : Gain  Gain=0.2
  IntegralTimeConstant : Constant  Value=AoyagiIntegralTimeConstant
  Integrator : Integrator  ExternalReset=either
  Integrator1 : Integrator  ExternalReset=either  LimitOutput=on  UpperSaturationLimit=20  LowerSaturationLimit=-20
  PhaseWrapper : LopesDevelopmentLibrary/Various/PhaseWrapper
  Saturation Dynamic : simulink/Discontinuities/Saturation Dynamic  OutMin=[]  OutMax=[]  OutDataTypeStr=Inherit: Same as second input  OutDataType=fixdt(1, 16)  OutScaling=2^-10  DoSatur=off
  Sum : Sum  Inputs=|+-
  Sum1 : Sum  Inputs=++|
  Sum2 : Sum  Inputs=++|
  ToPercentPerSec : Gain  Gain=100
  Wrap_Min50_Plus50 : Subsystem
  EstimatedPhase : Outport
  EstimatedPhaseRate : Outport  Port=2
  wires:
  ResetHighActive/1 -> Integrator1/2, Integrator/2
  Integrator/1 -> PhaseWrapper/1
  EstimatedPhaseUnfiltered/1 -> Sum/1
  Sum1/1 -> Saturation Dynamic/2
  AoyagiFilterGain/1 -> Sum1/2, Divide/2
  ToPercentPerSec/1 -> Sum2/2, Gain1/1, Gain/1
  PhaseWrapper/1 -> Sum/2, EstimatedPhase/1
  CalculateStridesPerSec/1 -> ToPercentPerSec/1
  Wrap_Min50_Plus50/1(Out) -> AoyagiFilterGain/1
  Saturation Dynamic/1 -> Integrator/1, EstimatedPhaseRate/1
  Sum/1 -> Wrap_Min50_Plus50/1(In)
  ReferenceStrideTime/1 -> CalculateStridesPerSec/1
  Gain1/1 -> Saturation Dynamic/3
  Gain/1 -> Saturation Dynamic/1
  IntegralTimeConstant/1 -> Divide/1
  Divide/1 -> Integrator1/1
  Integrator1/1 -> Sum2/1
  Sum2/1 -> Sum1/1
